simulink model "fourth"  (Simulink 7.4)
settings: Solver=ode23tb  StartTime=0.0  StopTime=1  MaxStep=1e-4  RelTol=1e-3
libraries: powerlib x7, powerlib_extras x3, aerolibutil x1
settings Model: Creator=lenovo  LastModifiedBy=lenovo
settings OptimizationCC: InitFltsAndDblsToZero=on
settings DebuggingCC: SaveWithParameterizedLinksMsg=none  SignalResolutionControl=TryResolveAllWithWarning  MultiTaskDSMMsg=warning  MultiTaskCondExecSysMsg=none
settings RTWCC: IncludeERTFirstTime=on
settings GRTTargetCC: TargetFcnLib=ansi_tfl_tmw.mat

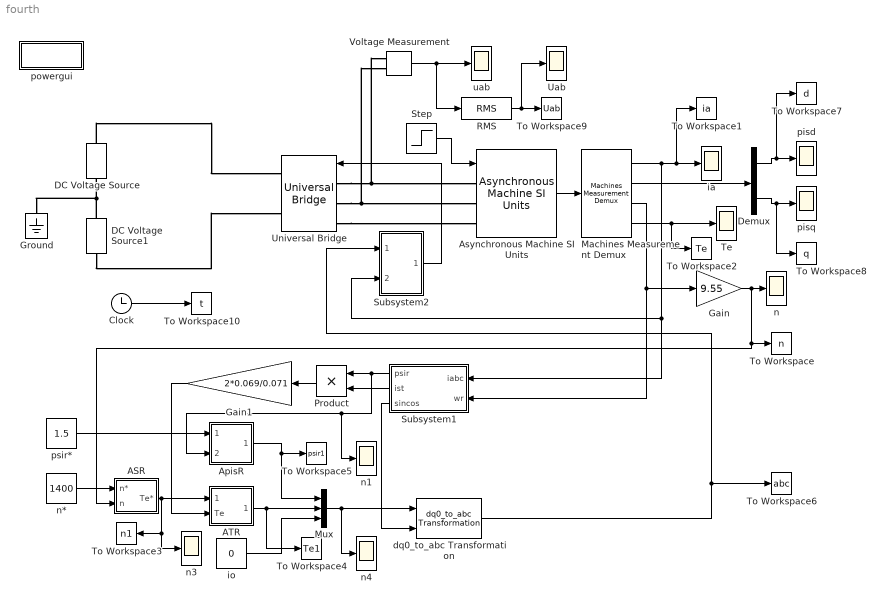
== system fourth ==
  ASR : Subsystem
  ATR : Subsystem
  ApisR : Subsystem
  Asynchronous Machine SI Units : powerlib/Machines/Asynchronous Machine SI Units  DialogController=POWERSYS.PowerSysDialog  SystemSampleTime=-1  PresetModel=No  MechanicalLoad=Torque Tm  ShowDetailedParameters=on  RotorType=Squirrel-cage  ReferenceFrame=Rotor  NominalParameters=[3730 380 50]  Stator=[0.435 0.002]  Rotor=[0.816 0.002]  Lm=0.069  Mechanical=[0.19 0.005752 2]  PolePairs=2  InitialConditions="[ 1,0   0,0,0   0,0,0 ]"  Units=SI  LoadFlowParameters=0  SimulateSaturation=off  Saturation=[9.9249,19.6672,38.0377,51.3988,69.2824,105.1337,152.5532,214.2421,303.1917;230, 322, 414, 460, 506, 552, 598, 644, 690]  TsPowergui=0  TsBlock=-1  IterativeModel=Forward Euler
  Clock : Clock
      settings: Decimation=10
  DC Voltage Source : powerlib/Electrical Sources/DC Voltage Source  DialogController=POWERSYS.PowerSysDialog  SystemSampleTime=-1  Amplitude=205  Measurements=None
  DC Voltage Source1 : powerlib/Electrical Sources/DC Voltage Source  DialogController=POWERSYS.PowerSysDialog  SystemSampleTime=-1  Amplitude=205  Measurements=None
  Demux : Demux  Outputs=2
  Gain : Gain  Gain=9.55  ParameterDataType=sfix(16)  ParameterScaling=2^0  OutDataType=sfix(16)  OutScaling=2^0
  Gain1 : Gain  Gain=2*0.069/0.071  ParameterDataType=sfix(16)  ParameterScaling=2^0  OutDataType=sfix(16)  OutScaling=2^0
  Ground : powerlib/Elements/Ground  DialogController=POWERSYS.PowerSysDialog  PhysicalDomain=powersysdomain  SubClassName=unknown  LeftPortType=p1  RightPortType=p1  LConnTagsString=a
  Machines Measurement Demux : powerlib/Machines/Machines Measurement Demux  DialogController=POWERSYS.PowerSysDialog  SystemSampleTime=-1  machType=Asynchronous  ssm1=on  ssm2=on  ssm3=on  ssm4=on  ssm5=on  ssm6=on  sm1=off  sm2=off  sm3=off  sm4=off  sm5=off  sm6=off  sm7=off  sm8=on  sm9=off  sm10=off  sm11=off  sm115=off  sm12=off  sm13=off  sm14=off  asm1=off  asm2=off  asm3=off  asm4=off  asm5=on  asm6=off  asm7=on  asm8=off  asm9=on  asm10=on  asm11=off  pmsm1=on  pmsm2=on  pmsm3=on  pmsm4=off  pmsm5=on  pmsm6=on  pmsm7=on  lastType=1
  Mux : Mux  Inputs=3
  Product : Product  OutDataType=sfix(16)  OutScaling=2^0  RndMeth=Zero
  RMS : powerlib_extras/Measurements/RMS  DialogController=POWERSYS.PowerSysDialog  SystemSampleTime=-1  f1=60
  Step : Step  Time=0.6  After=60  SampleTime=0
  Subsystem1 : Subsystem
  Subsystem2 : Subsystem
  Te : Scope
      settings: YMin=-1e-043  YMax=1.5e-042
  To Workspace : ToWorkspace  VariableName=n  SampleTime=-1  SaveFormat=Array
  To Workspace1 : ToWorkspace  VariableName=ia  SampleTime=-1  SaveFormat=Array
  To Workspace10 : ToWorkspace  VariableName=t  SampleTime=-1  SaveFormat=Array
  To Workspace2 : ToWorkspace  VariableName=Te  SampleTime=-1  SaveFormat=Array
  To Workspace3 : ToWorkspace  VariableName=n1  SampleTime=-1  SaveFormat=Array
  To Workspace4 : ToWorkspace  VariableName=Te1  SampleTime=-1  SaveFormat=Array
  To Workspace5 : ToWorkspace  VariableName=psir1  SampleTime=-1  SaveFormat=Array
  To Workspace6 : ToWorkspace  VariableName=abc  SampleTime=-1  SaveFormat=Array
  To Workspace7 : ToWorkspace  VariableName=d  SampleTime=-1  SaveFormat=Array
  To Workspace8 : ToWorkspace  VariableName=q  SampleTime=-1  SaveFormat=Array
  To Workspace9 : ToWorkspace  VariableName=Uab  SampleTime=-1  SaveFormat=Array
  Uab : Scope
      settings: YMin=-1  YMax=1  SaveName=ScopeData3
  Universal Bridge : powerlib/Power Electronics/Universal Bridge  DialogController=POWERSYS.PowerSysDialog  SystemSampleTime=-1  Arms=3  SnubberResistance=1e5  SnubberCapacitance=inf  Device=IGBT / Diodes  Ron=1e-3  Lon=0  ForwardVoltages="[  0  0  ]"  ForwardVoltage=0  GTOparameters=[ 10e-6 , 20e-6 ]  IGBTparameters=[ 1e-6 , 2e-6 ]  Measurements=None  Measurements_2=None  converterType=Rectifier
  Voltage Measurement : powerlib/Measurements/Voltage Measurement  DialogController=POWERSYS.PowerSysDialog  SystemSampleTime=-1  PhasorSimulation=off  OutputType=Complex  PSBequivalent=0
  dq0_to_abc Transformation : powerlib_extras/Measurements/dq0_to_abc Transformation  DialogController=POWERSYS.PowerSysDialog  SystemSampleTime=-1
  ia : Scope
  io : Constant  Value=0  OutDataType=sfix(16)  OutScaling=2^0
  n{,1,3..4} (4 alike) : Scope
      n settings: YMin=700  YMax=1450  SaveName=ScopeData2
      n1 settings: YMin=1.6e-005  YMax=2.8e-005  SaveName=ScopeData6
      n3 settings: YMin=71.25  YMax=78.75  SaveName=ScopeData8
      n4 settings: YMin=4.75e-007  YMax=5.55e-007  SaveName=ScopeData9
  n* : Constant  Value=1400  OutDataType=sfix(16)  OutScaling=2^0
  pisd : Scope
      settings: SaveName=d  DataFormat=Array
  pisq : Scope
      settings: SaveName=q  DataFormat=Array
  powergui : Subsystem  AncestorBlock=powerlib/powergui  InitFcn=|  mask(PSB option menu block){SimulationMode=Discrete, SampleTime=1e-4, echomessages=off, x0status=blocks, Frange=[0:2:500], Ylog=off, Xlog=on, ShowGrid=off, save=off, variable=ZData, structure=, ZoomFFT=on, StartTime=0.0, cycles=1, DisplayStyle=1, fundamental=60, FreqAxis=off, MaxFrequency=1000, frequencyindice=1, frequencyindicesteady=1, RmsSteady=1, display=off, Ts=0, frequency=60, methode=off}
      | powerguiblock = gcb;                                        
      | blk = get_param(powerguiblock,'blocks');                    
      | NbBlocks = length(blk);                                     
      | if NbBlocks>2                                               
      | % clean-up:                                                 
      | for m=1:NbBlocks-2                                          
      | delete_block([powerguiblock,'/EquivalentModel',num2str(m)]);
      | end                                                         
      | end
      mask prompts: SimulationMode "General parameter: Simulation Mode"; SampleTime "General parameter: Sample Time"; echomessages "General parameter: Echo  Messages"; x0status "Initial electrical states status"; Frange "Impedance tool: Frequency Range"; Ylog "Impedance tool: Log impedance"; Xlog "Impedance tool: log Frequency"; ShowGrid "Impedance tool: grid"; save "Impedance tool: Save Data To Workspace"; variable "Impedance tool: Variable Name"; structure "Structure Name (PSBFFTSCOPE)"; ZoomFFT "ZoomFFT (PSBFFTSCOPE)"; StartTime "Start Time (PSBFFTSCOPE)"; cycles "Cycles (PSBFFTSCOPE)"; DisplayStyle "Display style (PSBFFTSCOPE)"; fundamental "Fundamental (PSBFFTSCOPE)"; FreqAxis "Frequency Axis (PSBFFTSCOPE)"; MaxFrequency "Max Frequency (PSBFFTSCOPE)"; frequencyindice "Frequency indice  (PSBLOADFLOW)"; frequencyindicesteady "Frequency indice (STEADYSTATE)"; RmsSteady "RMS display (STEADYSTATE)"; display "Display Results"; Ts "Sample time (s):"; frequency "General parameter: phasor frequency"; methode "Phasor simulation"
      mask init:
      | powerlibroot = which('powersysdomain');
      | PSBroot = powerlibroot(1:end-16);
      | %
      | switch SimulationMode
      | 	case 1
      | 		message=sprintf('Continuous');
      | 	case 2
      |         message=sprintf('Discrete,\nTs = %.4g s.',SampleTime);
      | 	case 3
      | 		message=sprintf('Phasors');
      | end
      | if strcmp(bdroot,'powerlib')
      |   message='powergui';
      | end
      | power_initmask();
      settings: CopyFcn=powergui('Copy_Callback',gcb,0,[]);  DeleteFcn=powergui('Copy_Callback',gcb,1,[]);powergui('Close_Callback',gcb,[],[]);  ModelCloseFcn=powergui('Close_Callback',gcb,[],[]);  NameChangeFcn=handles = get_param(gcb,'UserData');if ~isempty(handles);delete(handles.powergui);end
      settings: PreSaveFcn=|
      | %try
      | %close(get_param(gcbh,'userdata'))
      | %end
      | 
      | powergui('Close_Callback',gcb,[],[]);
      settings: OpenFcn=|
      | if (power_openblockproxy ('secondary'))
      | powergui(gcb,'PM')
      | end;
      mask Help: web(psbhelp)
      mask StyleString: popup(Continuous|Discrete|Phasor),edit,checkbox,popup(blocks|steady|zero),edit,checkbox,checkbox,checkbox,checkbox,edit,edit,checkbox,edit,edit,edit,edit,checkbox,edit,edit,edit,edit,checkbox,edit,edit,checkbox
      mask Display: disp(message)
  psir* : Constant  Value=1.5  OutDataType=sfix(16)  OutScaling=2^0
  uab : Scope
      settings: YMin=-1  YMax=1  SaveName=ScopeData5
  wires:
  n*/1 -> ASR/1(n*)
  ASR/1(Te*) -> ATR/1(Te*), n3/1, To Workspace3/1
  ATR/1(ist*) -> Mux/2, To Workspace4/1
  io/1 -> Mux/3
  ApisR/1(ism*) -> Mux/1, To Workspace5/1
  psir*/1 -> ApisR/1(psir*)
  Mux/1 -> dq0_to_abc Transformation/1, n4/1
  Subsystem1/3(sincos) -> dq0_to_abc Transformation/2
  Subsystem1/2(ist) -> Product/2
  Subsystem1/1(psir) -> ApisR/2(psir), n1/1, Product/1
  Gain1/1 -> ATR/2(Te)
  Asynchronous Machine SI Units/1 -> Machines Measurement Demux/1
  Machines Measurement Demux/3 -> Subsystem1/2(wr), Gain/1
  Machines Measurement Demux/1 -> Subsystem1/1(iabc), Subsystem2/2(iabc), ia/1, To Workspace1/1
  Machines Measurement Demux/4 -> Te/1, To Workspace2/1
  Gain/1 -> n/1, ASR/2(n), To Workspace/1
  dq0_to_abc Transformation/1 -> Subsystem2/1(i*abc), To Workspace6/1
  Subsystem2/1(pulses) -> Universal Bridge/1
  Machines Measurement Demux/2 -> Demux/1
  Demux/1 -> pisd/1, To Workspace7/1
  Demux/2 -> pisq/1, To Workspace8/1
  Voltage Measurement/1 -> uab/1, RMS/1
  Step/1 -> Asynchronous Machine SI Units/1
  Product/1 -> Gain1/1
  RMS/1 -> To Workspace9/1, Uab/1
  Clock/1 -> To Workspace10/1
  connections:
  DC Voltage Source1/RConn1 -- DC Voltage Source/LConn1 -- Ground/LConn1
  Universal Bridge/LConn1 -- Asynchronous Machine SI Units/LConn1 -- Voltage Measurement/LConn1
  Universal Bridge/LConn2 -- Asynchronous Machine SI Units/LConn2 -- Voltage Measurement/LConn2
  Universal Bridge/LConn3 -- Asynchronous Machine SI Units/LConn3
  DC Voltage Source/RConn1 -- Universal Bridge/RConn1
  DC Voltage Source1/LConn1 -- Universal Bridge/RConn2

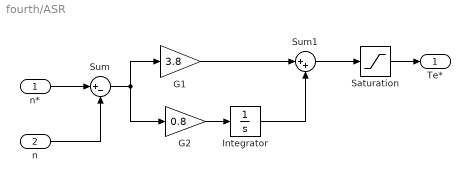
== system fourth/ASR ==
  n* : Inport  OutDataType=sfix(16)  OutScaling=2^0
  n : Inport  Port=2  OutDataType=sfix(16)  OutScaling=2^0
  G1 : Gain  Gain=3.8  ParameterDataType=sfix(16)  ParameterScaling=2^0  OutDataType=sfix(16)  OutScaling=2^0
  G2 : Gain  Gain=0.8  ParameterDataType=sfix(16)  ParameterScaling=2^0  OutDataType=sfix(16)  OutScaling=2^0
  Integrator : Integrator  LimitOutput=on  UpperSaturationLimit=80  LowerSaturationLimit=-80
  Saturation : Saturate  UpperLimit=75  LowerLimit=-75
  Sum : Sum  Inputs=|+-  OutDataType=sfix(16)  OutScaling=2^0
  Sum1 : Sum  Inputs=|++  OutDataType=sfix(16)  OutScaling=2^0
  Te* : Outport  OutDataType=sfix(16)  OutScaling=2^0
  wires:
  Saturation/1 -> Te*/1
  Sum1/1 -> Saturation/1
  Integrator/1 -> Sum1/2
  G1/1 -> Sum1/1
  G2/1 -> Integrator/1
  n/1 -> Sum/2
  Sum/1 -> G2/1, G1/1
  n*/1 -> Sum/1

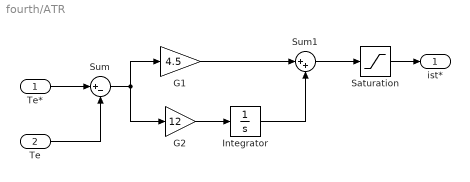
== system fourth/ATR ==
  Te* : Inport  OutDataType=sfix(16)  OutScaling=2^0
  Te : Inport  Port=2  OutDataType=sfix(16)  OutScaling=2^0
  G1 : Gain  Gain=4.5  ParameterDataType=sfix(16)  ParameterScaling=2^0  OutDataType=sfix(16)  OutScaling=2^0
  G2 : Gain  Gain=12  ParameterDataType=sfix(16)  ParameterScaling=2^0  OutDataType=sfix(16)  OutScaling=2^0
  Integrator : Integrator  LimitOutput=on  UpperSaturationLimit=60  LowerSaturationLimit=-60
  Saturation : Saturate  UpperLimit=60  LowerLimit=-60
  Sum : Sum  Inputs=|+-  OutDataType=sfix(16)  OutScaling=2^0
  Sum1 : Sum  Inputs=|++  OutDataType=sfix(16)  OutScaling=2^0
  ist* : Outport  OutDataType=sfix(16)  OutScaling=2^0
  wires:
  Saturation/1 -> ist*/1
  Sum1/1 -> Saturation/1
  Integrator/1 -> Sum1/2
  G1/1 -> Sum1/1
  G2/1 -> Integrator/1
  Te/1 -> Sum/2
  Sum/1 -> G2/1, G1/1
  Te*/1 -> Sum/1

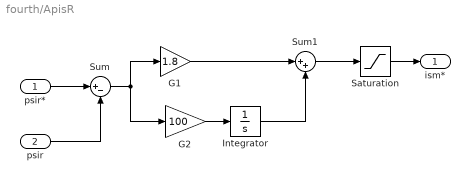
== system fourth/ApisR ==
  psir* : Inport  OutDataType=sfix(16)  OutScaling=2^0
  psir : Inport  Port=2  OutDataType=sfix(16)  OutScaling=2^0
  G1 : Gain  Gain=1.8  ParameterDataType=sfix(16)  ParameterScaling=2^0  OutDataType=sfix(16)  OutScaling=2^0
  G2 : Gain  Gain=100  ParameterDataType=sfix(16)  ParameterScaling=2^0  OutDataType=sfix(16)  OutScaling=2^0
  Integrator : Integrator  LimitOutput=on  UpperSaturationLimit=15  LowerSaturationLimit=-15
  Saturation : Saturate  UpperLimit=13  LowerLimit=-13
  Sum : Sum  Inputs=|+-  OutDataType=sfix(16)  OutScaling=2^0
  Sum1 : Sum  Inputs=|++  OutDataType=sfix(16)  OutScaling=2^0
  ism* : Outport  OutDataType=sfix(16)  OutScaling=2^0
  wires:
  Saturation/1 -> ism*/1
  Sum1/1 -> Saturation/1
  Integrator/1 -> Sum1/2
  G1/1 -> Sum1/1
  G2/1 -> Integrator/1
  psir/1 -> Sum/2
  Sum/1 -> G2/1, G1/1
  psir*/1 -> Sum/1

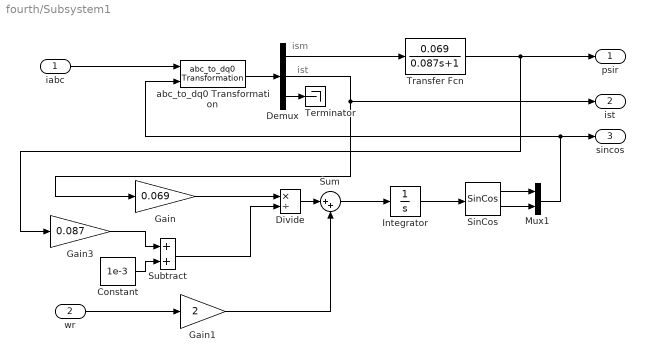
== system fourth/Subsystem1 ==
  note: ist
  note: ism
  iabc : Inport  OutDataType=sfix(16)  OutScaling=2^0
  wr : Inport  Port=2  OutDataType=sfix(16)  OutScaling=2^0
  Constant : Constant  Value=1e-3  OutDataType=sfix(16)  OutScaling=2^0
  Demux : Demux  Outputs=3
  Divide : Product  Inputs=*/  OutDataType=sfix(16)  OutScaling=2^-10
  Gain : Gain  Gain=0.069  ParameterDataType=sfix(16)  ParameterScaling=2^0  OutDataType=sfix(16)  OutScaling=2^0
  Gain1 : Gain  Gain=2  ParameterDataType=sfix(16)  ParameterScaling=2^0  OutDataType=sfix(16)  OutScaling=2^0
  Gain3 : Gain  Gain=0.087  ParameterDataType=sfix(16)  ParameterScaling=2^0  OutDataType=sfix(16)  OutScaling=2^0
  Integrator : Integrator
  Mux1 : Mux  Inputs=2
  SinCos : aerolibutil/SinCos  SystemSampleTime=-1
  Subtract : Sum  OutDataType=sfix(16)  OutScaling=2^-10
  Sum : Sum  Inputs=|++  OutDataType=sfix(16)  OutScaling=2^0
  Terminator : Terminator
  Transfer Fcn : TransferFcn  Numerator=[0.069]  Denominator=[0.087 1]
  abc_to_dq0 Transformation : powerlib_extras/Measurements/abc_to_dq0 Transformation  DialogController=POWERSYS.PowerSysDialog  SystemSampleTime=-1
  psir : Outport  OutDataType=sfix(16)  OutScaling=2^0
  ist : Outport  Port=2  OutDataType=sfix(16)  OutScaling=2^0
  sincos : Outport  Port=3  OutDataType=sfix(16)  OutScaling=2^0
  wires:
  Mux1/1 -> abc_to_dq0 Transformation/2, sincos/1
  SinCos/2 -> Mux1/2
  SinCos/1 -> Mux1/1
  Demux/3 -> Terminator/1
  Demux/2 -> ist/1, Gain/1
  Integrator/1 -> SinCos/1
  Sum/1 -> Integrator/1
  Gain1/1 -> Sum/2
  wr/1 -> Gain1/1
  Transfer Fcn/1 -> psir/1, Gain3/1
  Demux/1 -> Transfer Fcn/1
  abc_to_dq0 Transformation/1 -> Demux/1
  iabc/1 -> abc_to_dq0 Transformation/1
  Gain/1 -> Divide/1
  Subtract/1 -> Divide/2
  Constant/1 -> Subtract/2
  Gain3/1 -> Subtract/1
  Divide/1 -> Sum/1

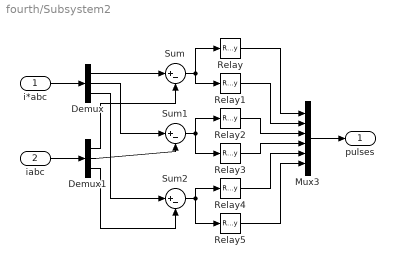
== system fourth/Subsystem2 ==
  i*abc : Inport  OutDataType=sfix(16)  OutScaling=2^0
  iabc : Inport  Port=2  OutDataType=sfix(16)  OutScaling=2^0
  Demux : Demux  Outputs=3
  Demux1 : Demux  Outputs=3
  Mux3 : Mux  Inputs=6
  Relay : Relay  OnSwitchValue=0.5  OffSwitchValue=-0.5  OutDataType=sfix(16)  OutScaling=2^0
  Relay1 : Relay  OnSwitchValue=0.5  OffSwitchValue=-0.5  OnOutputValue=0  OffOutputValue=1  OutDataType=sfix(16)  OutScaling=2^0
  Relay2 : Relay  OnSwitchValue=0.5  OffSwitchValue=-0.5  OutDataType=sfix(16)  OutScaling=2^0
  Relay3 : Relay  OnSwitchValue=0.5  OffSwitchValue=-0.5  OnOutputValue=0  OffOutputValue=1  OutDataType=sfix(16)  OutScaling=2^0
  Relay4 : Relay  OnSwitchValue=0.5  OffSwitchValue=-0.5  OutDataType=sfix(16)  OutScaling=2^0
  Relay5 : Relay  OnSwitchValue=0.5  OffSwitchValue=-0.5  OnOutputValue=0  OffOutputValue=1  OutDataType=sfix(16)  OutScaling=2^0
  Sum : Sum  Inputs=|+-  OutDataType=sfix(16)  OutScaling=2^0
  Sum1 : Sum  Inputs=|+-  OutDataType=sfix(16)  OutScaling=2^0
  Sum2 : Sum  Inputs=|+-  OutDataType=sfix(16)  OutScaling=2^0
  pulses : Outport  OutDataType=sfix(16)  OutScaling=2^0
  wires:
  Mux3/1 -> pulses/1
  Relay5/1 -> Mux3/6
  Relay4/1 -> Mux3/5
  Relay3/1 -> Mux3/4
  Relay2/1 -> Mux3/3
  Relay1/1 -> Mux3/2
  Relay/1 -> Mux3/1
  Sum2/1 -> Relay4/1, Relay5/1
  Sum1/1 -> Relay3/1, Relay2/1
  Sum/1 -> Relay1/1, Relay/1
  Demux1/3 -> Sum2/2
  Demux1/2 -> Sum1/2
  Demux1/1 -> Sum/2
  Demux/3 -> Sum2/1
  Demux/2 -> Sum1/1
  Demux/1 -> Sum/1
  iabc/1 -> Demux1/1
  i*abc/1 -> Demux/1

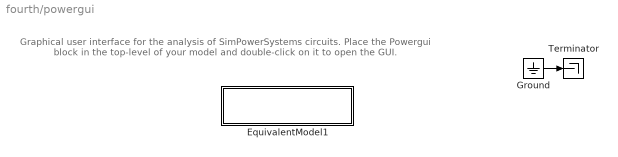
== system fourth/powergui ==
  note: Graphical user interface for the analysis of  SimPowerSystems circuits.
      | Place the Powergui block in the top-level of your model and double-click
      | on it to open the GUI.
  EquivalentModel1 : Subsystem
      mask init:
      | SPS = get_param(gcbh,'UserData');
      | if isempty(SPS)
      | 	Ts=1;
      |     A=0;
      |     B=0;
      |     C=0;
      |     D=0;
      |     x0=0;
      |     SwitchResistance=1;
      |     SwitchType=1;
      |     SwitchGateInitialValue=1;
      |     OutputsToResetToZero=1;
      | else
      | 	Ts=SPS.fixedstep;
      | 	A=SPS.Adiscrete;
      |     B=SPS.Bdiscrete;
      |     C=SPS.Cdiscrete;
      |     D=SPS.Ddiscrete;
      |     x0=SPS.x0discrete;
      |     SwitchResistance=SPS.SwitchResistance;
      |     SwitchType=SPS.SwitchType;
      |     SwitchGateInitialValue=SPS.SwitchGateInitialValue;
      |     OutputsToResetToZero=SPS.YSwitchCurrent;
      | end
      mask Display:
      | color('orange')
      | disp('EQUIVALENT CIRCUIT')
  Ground : Ground
  Terminator : Terminator
  wires:
  Ground/1 -> Terminator/1

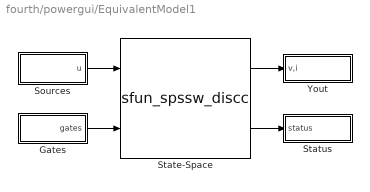
== system fourth/powergui/EquivalentModel1 ==
  Gates : Subsystem
  Sources : Subsystem
  State-Space : S-Function  FunctionName=sfun_spssw_discc  Parameters=Ts,A, B, C, D, x0, SwitchResistance ,SwitchType, SwitchGateInitialValue, OutputsToResetToZero  EnableBusSupport=off
  Status : Subsystem
  Yout : Subsystem
  wires:
  Gates/1(gates) -> State-Space/2
  Sources/1(u) -> State-Space/1
  State-Space/2 -> Status/1(status)
  State-Space/1 -> Yout/1(v,i)

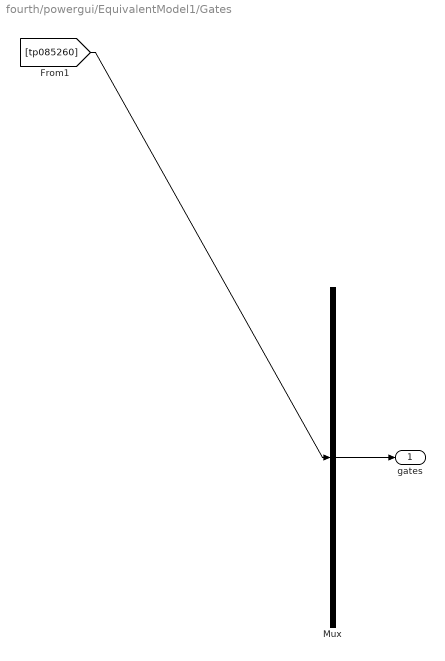
== system fourth/powergui/EquivalentModel1/Gates ==
  Mux : Mux  Inputs=1
  gates : Outport  OutDataType=sfix(16)  OutScaling=2^0
  wires:
  Mux/1 -> gates/1
  [tp085260] -> Mux/1

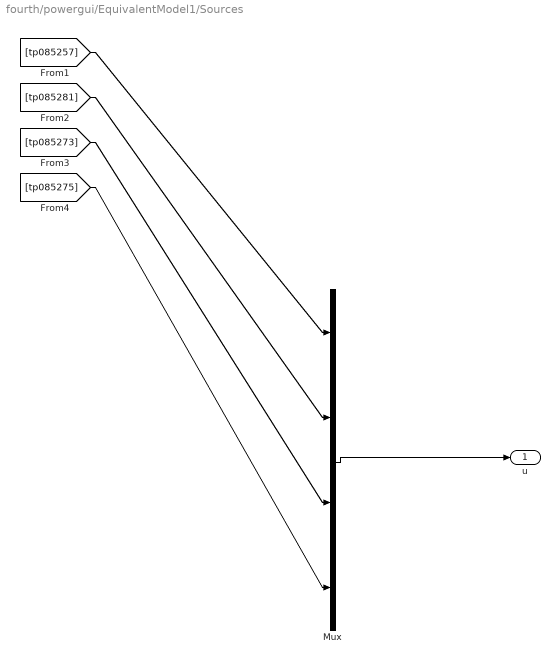
== system fourth/powergui/EquivalentModel1/Sources ==
  Mux : Mux  Inputs=[6 2 1 1]
  u : Outport  OutDataType=sfix(16)  OutScaling=2^0
  wires:
  Mux/1 -> u/1
  [tp085257] -> Mux/1
  [tp085281] -> Mux/2
  [tp085273] -> Mux/3
  [tp085275] -> Mux/4

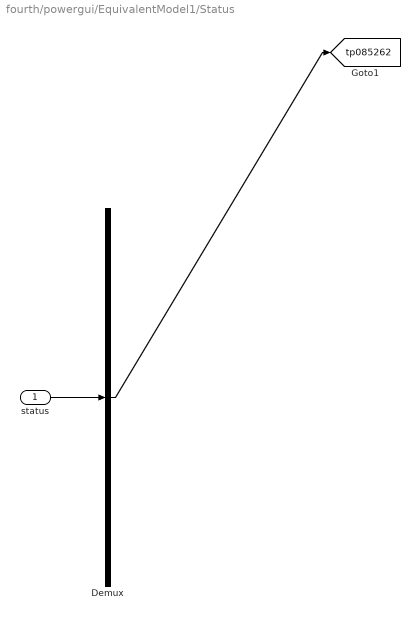
== system fourth/powergui/EquivalentModel1/Status ==
  status : Inport  OutDataType=sfix(16)  OutScaling=2^0
  Demux : Demux  Outputs=1
  tag scope: tp085262=global
  wires:
  status/1 -> Demux/1
  Demux/1 -> [tp085262]

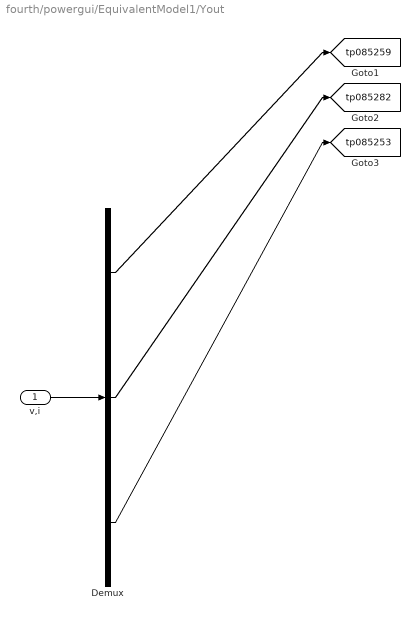
== system fourth/powergui/EquivalentModel1/Yout ==
  v,i : Inport  OutDataType=sfix(16)  OutScaling=2^0
  Demux : Demux  Outputs=[6 2 1]
  tag scope: tp085253=global, tp085259=global, tp085282=global
  wires:
  v,i/1 -> Demux/1
  Demux/1 -> [tp085259]
  Demux/2 -> [tp085282]
  Demux/3 -> [tp085253]
